simulink library "cdsOsc"  (Simulink 7.2)
settings: Solver=ode45  SolverMode=SingleTasking  StartTime=0.0  StopTime=10.0  RelTol=1e-3
settings Model: Creator=maronsso  LastModifiedBy=rolf

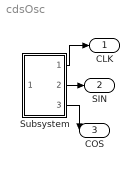
== system cdsOsc ==
  Subsystem : Subsystem
  CLK : Outport
  SIN : Outport  Port=2
  COS : Outport  Port=3
  wires:
  Subsystem/1(CLK) -> CLK/1
  Subsystem/2(SIN) -> SIN/1
  Subsystem/3(COS) -> COS/1

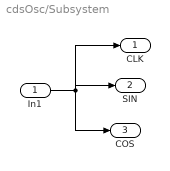
== system cdsOsc/Subsystem ==
  In1 : Inport  OutDataType=sfix(16)  OutScaling=2^0
  CLK : Outport  OutDataType=sfix(16)  OutScaling=2^0
  SIN : Outport  Port=2  OutDataType=sfix(16)  OutScaling=2^0
  COS : Outport  Port=3  OutDataType=sfix(16)  OutScaling=2^0
  wires:
  In1/1 -> CLK/1, SIN/1, COS/1
